simulink model "Control_motores"  (R2025b)
settings: Solver=VariableStepAuto  StartTime=0.0  StopTime=2  RelTol=1e-3
settings Model: Creator=ASUS TUF  LastModifiedBy=ASUS TUF

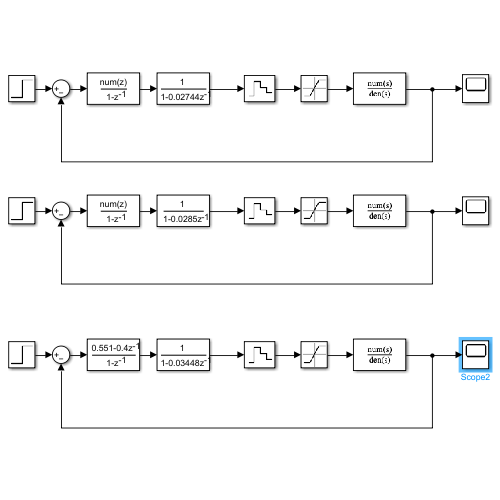
[thumbnail: Simulink's stored preview of the top-level diagram]
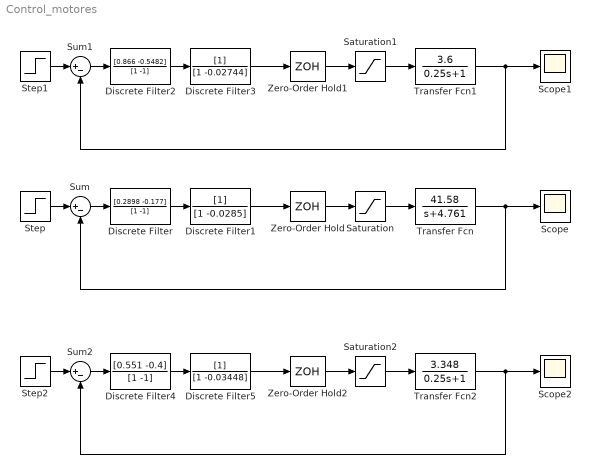
== system Control_motores ==
  Discrete Filter : DiscreteFilter  Numerator=[0.2898 -0.177]  Denominator=[1 -1]
  Discrete Filter1 : DiscreteFilter  Denominator=[1 -0.0285]
  Discrete Filter2 : DiscreteFilter  Numerator=[0.866 -0.5482]  Denominator=[1 -1]
  Discrete Filter3 : DiscreteFilter  Denominator=[1 -0.02744]
  Discrete Filter4 : DiscreteFilter  Numerator=[0.551 -0.4]  Denominator=[1 -1]
  Discrete Filter5 : DiscreteFilter  Denominator=[1 -0.03448]
  Saturation : Saturate  UpperLimit=12  LowerLimit=-12
  Saturation1 : Saturate  UpperLimit=12  LowerLimit=-12
  Saturation2 : Saturate  UpperLimit=12  LowerLimit=-12
  Scope : Scope
      settings: ActiveDisplayYMinimum=-1.433184376299977  ActiveDisplayYMaximum=12.898659386699794
  Scope1 : Scope
      settings: ActiveDisplayYMinimum=-1.4605849132339523  ActiveDisplayYMaximum=13.145264219105574
  Scope2 : Scope
      settings: ActiveDisplayYMinimum=-1.3371184689005384  ActiveDisplayYMaximum=12.034066220104847  DataLoggingVariableName=ScopeData2
  Step : Step  Time=0  After=10  SampleTime=0
  Step1 : Step  Time=0  After=10  SampleTime=0
  Step2 : Step  Time=0  After=10  SampleTime=0
  Sum : Sum  Inputs=|+-
  Sum1 : Sum  Inputs=|+-
  Sum2 : Sum  Inputs=|+-
  Transfer Fcn : TransferFcn  Numerator=[41.58]  Denominator=[1 4.761]
  Transfer Fcn1 : TransferFcn  Numerator=[3.6]  Denominator=[0.25 1]
  Transfer Fcn2 : TransferFcn  Numerator=[3.348]  Denominator=[0.25 1]
  Zero-Order Hold : ZeroOrderHold  SampleTime=0.05
  Zero-Order Hold1 : ZeroOrderHold  SampleTime=0.05
  Zero-Order Hold2 : ZeroOrderHold  SampleTime=0.05
  wires:
  Transfer Fcn/1 -> Sum/2, Scope/1
  Step/1 -> Sum/1
  Sum/1 -> Discrete Filter/1
  Discrete Filter/1 -> Discrete Filter1/1
  Discrete Filter1/1 -> Zero-Order Hold/1
  Saturation/1 -> Transfer Fcn/1
  Zero-Order Hold/1 -> Saturation/1
  Zero-Order Hold1/1 -> Saturation1/1
  Discrete Filter3/1 -> Zero-Order Hold1/1
  Discrete Filter2/1 -> Discrete Filter3/1
  Step1/1 -> Sum1/1
  Saturation1/1 -> Transfer Fcn1/1
  Transfer Fcn1/1 -> Sum1/2, Scope1/1
  Sum1/1 -> Discrete Filter2/1
  Zero-Order Hold2/1 -> Saturation2/1
  Discrete Filter5/1 -> Zero-Order Hold2/1
  Discrete Filter4/1 -> Discrete Filter5/1
  Step2/1 -> Sum2/1
  Saturation2/1 -> Transfer Fcn2/1
  Transfer Fcn2/1 -> Sum2/2, Scope2/1
  Sum2/1 -> Discrete Filter4/1
